simulink model "system1"  (R2018b)
settings: Solver=VariableStepAuto  StartTime=0.0  StopTime=20  RelTol=1e-3
libraries: cstblocks x3, simulink x1
settings Model: Creator=Abraham Pérez  LastModifiedBy=Abraham Pérez

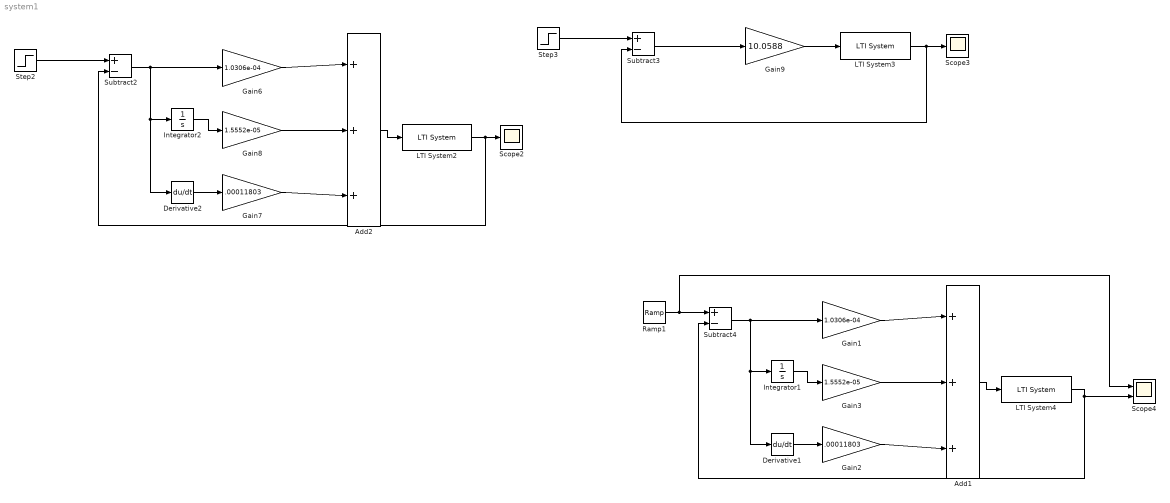
== system system1 ==
  Add1 : Sum  Inputs=+++
  Add2 : Sum  Inputs=+++
  Derivative1 : Derivative
  Derivative2 : Derivative
  Gain1 : Gain  Gain=1.0306e-04
  Gain2 : Gain  Gain=.00011803
  Gain3 : Gain  Gain=1.5552e-05
  Gain6 : Gain  Gain=1.0306e-04
  Gain7 : Gain  Gain=.00011803
  Gain8 : Gain  Gain=1.5552e-05
  Gain9 : Gain  Gain=10.0588
  Integrator1 : Integrator
  Integrator2 : Integrator
  LTI System2 : cstblocks/LTI System  sys=G1  IC=[]
  LTI System3 : cstblocks/LTI System  sys=G1  IC=[]
  LTI System4 : cstblocks/LTI System  sys=G1  IC=[]
  Ramp1 : simulink/Sources/Ramp  slope=1  start=0  InitialOutput=17
  Scope2 : Scope
  Scope3 : Scope
  Scope4 : Scope  NumInputPorts=2
  Step2 : Step  Time=0  After=9  SampleTime=0
  Step3 : Step  Time=0  SampleTime=0
  Subtract2 : Sum  Inputs=+-
  Subtract3 : Sum  Inputs=+-
  Subtract4 : Sum  Inputs=+-
  wires:
  Add2/1 -> LTI System2/1
  Subtract2/1 -> Derivative2/1, Integrator2/1, Gain6/1
  Gain8/1 -> Add2/2
  Integrator2/1 -> Gain8/1
  Step2/1 -> Subtract2/1
  Gain6/1 -> Add2/1
  Gain7/1 -> Add2/3
  Derivative2/1 -> Gain7/1
  LTI System2/1 -> Subtract2/2, Scope2/1
  LTI System3/1 -> Subtract3/2, Scope3/1
  Step3/1 -> Subtract3/1
  Subtract3/1 -> Gain9/1
  Gain9/1 -> LTI System3/1
  Subtract4/1 -> Derivative1/1, Integrator1/1, Gain1/1
  Derivative1/1 -> Gain2/1
  Gain3/1 -> Add1/2
  Gain2/1 -> Add1/3
  LTI System4/1 -> Subtract4/2, Scope4/2
  Add1/1 -> LTI System4/1
  Integrator1/1 -> Gain3/1
  Gain1/1 -> Add1/1
  Ramp1/1 -> Scope4/1, Subtract4/1
